simulink model "BACKSTEPPING_ULTIMAVERSION"  (R2024b)
settings: Solver=VariableStepAuto  StartTime=0.0  StopTime=100  RelTol=1e-3
libraries: simulink x1
settings Model: Creator=LENOVO  LastModifiedBy=aliss
settings SolverCC: AlgebraicLoopSolver=TrustRegion
settings DebuggingCC: UnconnectedInputMsg=warning  UnconnectedOutputMsg=warning  UnconnectedLineMsg=warning
settings ModelReferenceCC: EnableRefExpFcnMdlSchedulingChecks=on
settings RTWCC: GPUComputeCapability=3.5

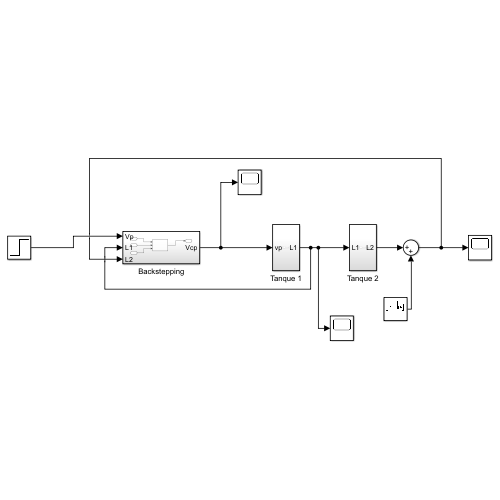
[thumbnail: Simulink's stored preview of the top-level diagram]
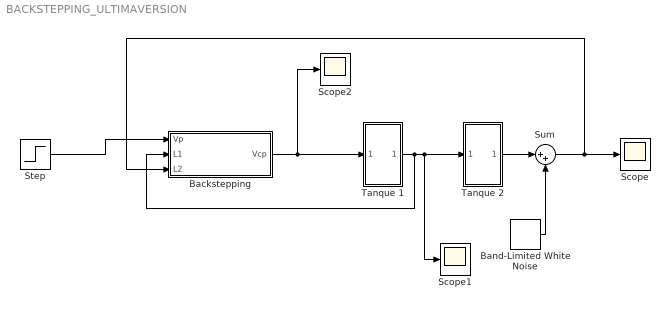
== system BACKSTEPPING_ULTIMAVERSION ==
  Backstepping : Subsystem
  Band-Limited White Noise : simulink/Sources/Band-Limited White Noise  Cov=[0.1]  Ts=5  seed=[23341]
  Scope : Scope
  Scope1 : Scope
  Scope2 : Scope
  Step : Step  After=6  SampleTime=0
  Sum : Sum  Inputs=|++
  Tanque 1 : Subsystem
  Tanque 2 : Subsystem
  wires:
  Tanque 1/1(L1) -> Backstepping/2(L1), Scope1/1, Tanque 2/1(L1)
  Backstepping/1(Vcp) -> Scope2/1, Tanque 1/1(vp)
  Step/1 -> Backstepping/1(Vp)
  Tanque 2/1(L2) -> Sum/1
  Sum/1 -> Backstepping/3(L2), Scope/1
  Band-Limited White Noise/1 -> Sum/2

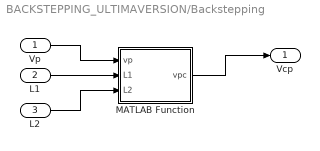
== system BACKSTEPPING_ULTIMAVERSION/Backstepping ==
  Vp : Inport
  L1 : Inport  Port=2
  L2 : Inport  Port=3
  MATLAB Function : MATLAB Function  TreatAsAtomicUnit=on
  Vcp : Outport
  wires:
  Vp/1 -> MATLAB Function/1(vp)
  MATLAB Function/1(vpc) -> Vcp/1
  L2/1 -> MATLAB Function/3(L2)
  L1/1 -> MATLAB Function/2(L1)

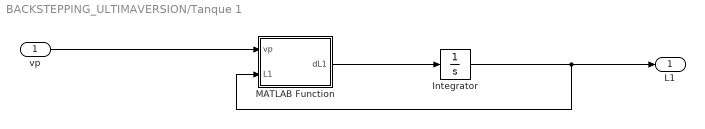
== system BACKSTEPPING_ULTIMAVERSION/Tanque 1 ==
  vp : Inport
  Integrator : Integrator
  MATLAB Function : MATLAB Function  TreatAsAtomicUnit=on
  L1 : Outport
  wires:
  Integrator/1 -> L1/1, MATLAB Function/2(L1)
  MATLAB Function/1(dL1) -> Integrator/1
  vp/1 -> MATLAB Function/1(vp)

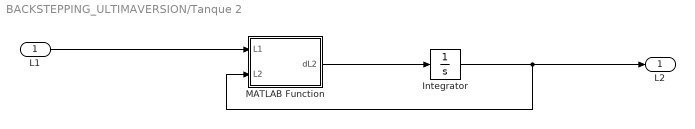
== system BACKSTEPPING_ULTIMAVERSION/Tanque 2 ==
  L1 : Inport
  Integrator : Integrator
  MATLAB Function : MATLAB Function  TreatAsAtomicUnit=on
  L2 : Outport
  wires:
  Integrator/1 -> MATLAB Function/2(L2), L2/1
  MATLAB Function/1(dL2) -> Integrator/1
  L1/1 -> MATLAB Function/1(L1)

== matlab function BACKSTEPPING_ULTIMAVERSION/Tanque 2/MATLAB Function ==
  data: L1 input; L2 input; dL2 output
function dL2 = fcn(L1, L2)
if L2<0 
   L2=0; 
end
d1=0.635;
a1=pi*d1^2/4;
D2=4.445;
d2=0.47625;
A2=pi*D2^2/4;
a2=pi*d2^2/4;
g=980;

Qin=sqrt(2*g*L1)*a1;
Vout2=sqrt(2*g*L2);
Qout2=Vout2*a2;

dL2 = (Qin-Qout2)/A2;

== matlab function BACKSTEPPING_ULTIMAVERSION/Tanque 1/MATLAB Function ==
  data: vp input; dL1 output; L1 input
function dL1 = fcn(vp, L1)

D1=4.445;
d1=0.635;
A1=pi*D1^2/4;
a1=pi*d1^2/4;
Kp=3.3;
g=980;

Qi=vp*Kp;
Vout=sqrt(2*g*L1);
Qout=Vout*a1;

dL1 = (Qi-Qout)/A1;

== matlab function BACKSTEPPING_ULTIMAVERSION/Backstepping/MATLAB Function ==
  data: vp input; vpc output; L1 input; L2 input
function vpc = fcn(vp,L1,L2)

x1=L2;
x2=L1;
h2d=3;

c1=3;
c2=2;

D1=4.445;
d1=0.635;
A1=pi*D1^2/4;
a1=pi*d1^2/4;
Kp=3.3;
g=980;

D2=4.445;
d2=0.47625;
A2=pi*D2^2/4;
a2=pi*d2^2/4;

B=a1*sqrt(2*g)/A2;
B2=a2*sqrt(2*g)/A2;

y=Kp/A1;
y2=a1*sqrt(2*g)/A1;

if L2<h2d
    vpc=vp;
else

    z1=x1-h2d;
    phi=(B2*sqrt(x1)-c1*z1)/B;
    z2=sqrt(x2)-phi;

    dphi=((B2/2*sqrt(x1)-c1)*(B*sqrt(x2)-B2*sqrt(x1)))/B;
    u=(2*sqrt(x2)*(dphi-c2*z2-B*z1+y2/2))/y;
    if u<=-vp
        vpc=0;
    else
        vpc=vp+u;
    end
end
